simulink model "mdl_Noramlized_LPF_SAR_parallel"  (R2023b)
settings: Solver=VariableStepAuto  StartTime=0.0  StopTime=T_run  FixedStep=1/2.048e6  MaxStep=1e-8  MinStep=1e-12  RelTol=1e-5
undefined symbols (not defined in the file or in its folder): delay, f_s, f_sig, H_matrix, k, NOB, osr, pulse_width, seed_offset, VFS, Vrms
libraries: simulink x9, simulink_extras x8, dspsigops x8
settings Model: Creator=prest  LastModifiedBy=Adyant Balaji
settings DebuggingCC: UnconnectedInputMsg=warning  UnconnectedOutputMsg=warning  UnconnectedLineMsg=warning
settings ModelReferenceCC: EnableRefExpFcnMdlSchedulingChecks=on
settings RTWCC: DLArmComputeVersion=19.05

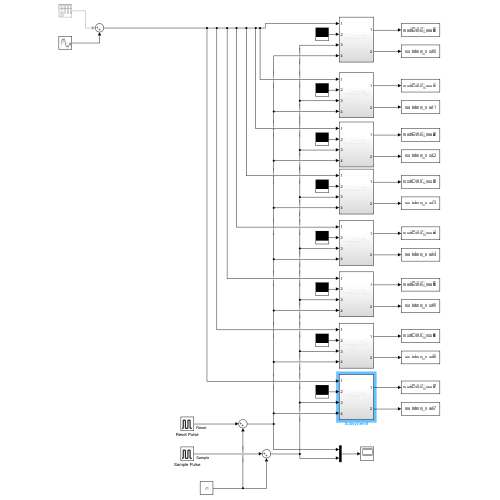
[thumbnail: Simulink's stored preview of the top-level diagram]
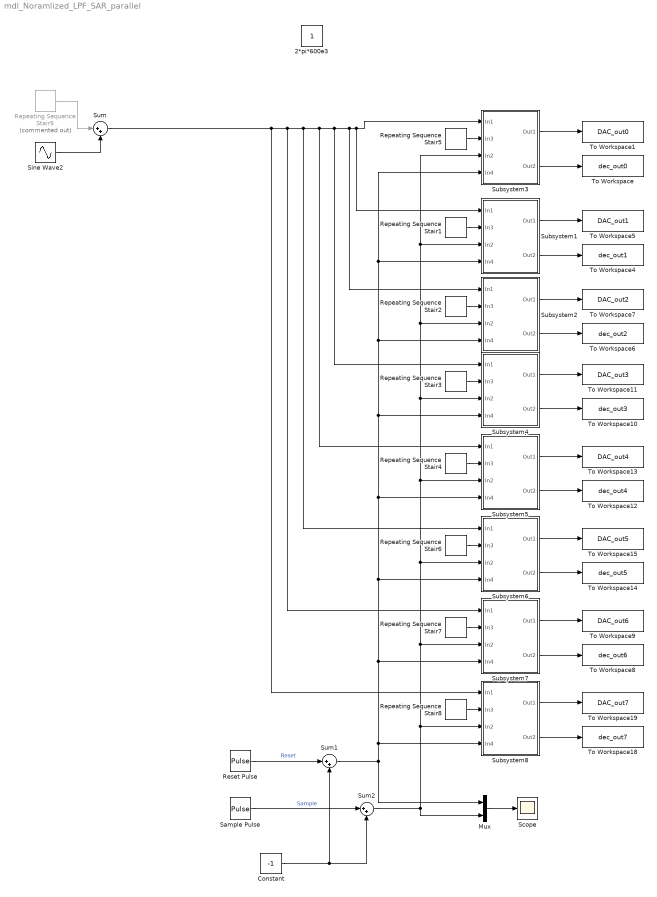
== system mdl_Noramlized_LPF_SAR_parallel ==
  Constant : Constant  Value=-1
  Mux : Mux  Inputs=2
  Repeating Sequence Stair1 : simulink/Sources/Repeating Sequence Stair  OutValues=H_matrix(:, k+1)  tsamp=T_hadamard  OutMin=[]  OutMax=[]  OutDataTypeStr=double  OutputDataTypeScalingMode=double  OutDataType=fixdt(0,8)  ConRadixGroup=Best Precision: Vector-wise  OutScaling=2^-12
  Repeating Sequence Stair2 : simulink/Sources/Repeating Sequence Stair  OutValues=H_matrix(:, k+2)  tsamp=T_hadamard  OutMin=[]  OutMax=[]  OutDataTypeStr=double  OutputDataTypeScalingMode=double  OutDataType=fixdt(0,8)  ConRadixGroup=Best Precision: Vector-wise  OutScaling=2^-12
  Repeating Sequence Stair3 : simulink/Sources/Repeating Sequence Stair  OutValues=H_matrix(:, k+3)  tsamp=T_hadamard  OutMin=[]  OutMax=[]  OutDataTypeStr=double  OutputDataTypeScalingMode=double  OutDataType=fixdt(0,8)  ConRadixGroup=Best Precision: Vector-wise  OutScaling=2^-12
  Repeating Sequence Stair4 : simulink/Sources/Repeating Sequence Stair  OutValues=H_matrix(:, k+4)  tsamp=T_hadamard  OutMin=[]  OutMax=[]  OutDataTypeStr=double  OutputDataTypeScalingMode=double  OutDataType=fixdt(0,8)  ConRadixGroup=Best Precision: Vector-wise  OutScaling=2^-12
  Repeating Sequence Stair5 : simulink/Sources/Repeating Sequence Stair  OutValues=H_matrix(:, k)  tsamp=T_hadamard  OutMin=[]  OutMax=[]  OutDataTypeStr=double  OutputDataTypeScalingMode=double  OutDataType=fixdt(0,8)  ConRadixGroup=Best Precision: Vector-wise  OutScaling=2^-12
  Repeating Sequence Stair6 : simulink/Sources/Repeating Sequence Stair  OutValues=H_matrix(:, k+5)  tsamp=T_hadamard  OutMin=[]  OutMax=[]  OutDataTypeStr=double  OutputDataTypeScalingMode=double  OutDataType=fixdt(0,8)  ConRadixGroup=Best Precision: Vector-wise  OutScaling=2^-12
  Repeating Sequence Stair7 : simulink/Sources/Repeating Sequence Stair  OutValues=H_matrix(:, k+6)  tsamp=T_hadamard  OutMin=[]  OutMax=[]  OutDataTypeStr=double  OutputDataTypeScalingMode=double  OutDataType=fixdt(0,8)  ConRadixGroup=Best Precision: Vector-wise  OutScaling=2^-12
  Repeating Sequence Stair8 : simulink/Sources/Repeating Sequence Stair  OutValues=H_matrix(:, k+7)  tsamp=T_hadamard  OutMin=[]  OutMax=[]  OutDataTypeStr=double  OutputDataTypeScalingMode=double  OutDataType=fixdt(0,8)  ConRadixGroup=Best Precision: Vector-wise  OutScaling=2^-12
  Repeating Sequence Stair9 : simulink/Sources/Repeating Sequence Stair  Commented=on  OutValues=input_sequence  tsamp=T_hadamard  OutMin=[]  OutMax=[]  OutDataTypeStr=double  OutputDataTypeScalingMode=double  OutDataType=fixdt(0,8)  ConRadixGroup=Best Precision: Vector-wise  OutScaling=2^-12
  Reset Pulse : DiscretePulseGenerator  PulseType=Time based  Amplitude=2  Period=osr/f_s  PulseWidth=pulse_width  PhaseDelay=delay
  Sample Pulse : DiscretePulseGenerator  PulseType=Time based  Amplitude=2  Period=osr/f_s  PulseWidth=0.001
  Scope : Scope
  Sine Wave2 : Sin  Amplitude=VFS/2-0.05  Frequency=2*pi*f_sig  SampleTime=0
  Subsystem1 : Subsystem
  Subsystem2 : Subsystem
  Subsystem3 : Subsystem
  Subsystem4 : Subsystem
  Subsystem5 : Subsystem
  Subsystem6 : Subsystem
  Subsystem7 : Subsystem
  Subsystem8 : Subsystem
  Sum : Sum  Inputs=|++
  Sum1 : Sum  Inputs=|++
  Sum2 : Sum  Inputs=|++
  To Workspace : ToWorkspace  VariableName=dec_out0  SampleTime=-1
  To Workspace1 : ToWorkspace  VariableName=DAC_out0  SampleTime=-1
  To Workspace10 : ToWorkspace  VariableName=dec_out3  SampleTime=-1
  To Workspace11 : ToWorkspace  VariableName=DAC_out3  SampleTime=-1
  To Workspace12 : ToWorkspace  VariableName=dec_out4  SampleTime=-1
  To Workspace13 : ToWorkspace  VariableName=DAC_out4  SampleTime=-1
  To Workspace14 : ToWorkspace  VariableName=dec_out5  SampleTime=-1
  To Workspace15 : ToWorkspace  VariableName=DAC_out5  SampleTime=-1
  To Workspace18 : ToWorkspace  VariableName=dec_out7  SampleTime=-1
  To Workspace19 : ToWorkspace  VariableName=DAC_out7  SampleTime=-1
  To Workspace4 : ToWorkspace  VariableName=dec_out1  SampleTime=-1
  To Workspace5 : ToWorkspace  VariableName=DAC_out1  SampleTime=-1
  To Workspace6 : ToWorkspace  VariableName=dec_out2  SampleTime=-1
  To Workspace7 : ToWorkspace  VariableName=DAC_out2  SampleTime=-1
  To Workspace8 : ToWorkspace  VariableName=dec_out6  SampleTime=-1
  To Workspace9 : ToWorkspace  VariableName=DAC_out6  SampleTime=-1
  2*pi*600e3 : Constant  IOType=siggen
  wires:
  Sum/1 -> Subsystem8/1(In1), Subsystem7/1(In1), Subsystem6/1(In1), Subsystem5/1(In1), Subsystem4/1(In1), Subsystem2/1(In1), Subsystem1/1(In1), Subsystem3/1(In1)
  Repeating Sequence Stair5/1 -> Subsystem3/2(In3)
  Subsystem3/1(Out1) -> To Workspace1/1
  Subsystem3/2(Out2) -> To Workspace/1
  Repeating Sequence Stair1/1 -> Subsystem1/2(In3)
  Repeating Sequence Stair8/1 -> Subsystem8/2(In3)
  Subsystem2/2(Out2) -> To Workspace6/1
  Subsystem2/1(Out1) -> To Workspace7/1
  Subsystem1/1(Out1) -> To Workspace5/1
  Subsystem1/2(Out2) -> To Workspace4/1
  Subsystem7/1(Out1) -> To Workspace9/1
  Subsystem7/2(Out2) -> To Workspace8/1
  Subsystem5/1(Out1) -> To Workspace13/1
  Subsystem6/2(Out2) -> To Workspace14/1
  Subsystem6/1(Out1) -> To Workspace15/1
  Subsystem4/2(Out2) -> To Workspace10/1
  Subsystem4/1(Out1) -> To Workspace11/1
  Subsystem5/2(Out2) -> To Workspace12/1
  Subsystem8/2(Out2) -> To Workspace18/1
  Subsystem8/1(Out1) -> To Workspace19/1
  Repeating Sequence Stair2/1 -> Subsystem2/2(In3)
  Repeating Sequence Stair3/1 -> Subsystem4/2(In3)
  Repeating Sequence Stair4/1 -> Subsystem5/2(In3)
  Repeating Sequence Stair6/1 -> Subsystem6/2(In3)
  Repeating Sequence Stair7/1 -> Subsystem7/2(In3)
  Repeating Sequence Stair9/1 -> Sum/1
  Sine Wave2/1 -> Sum/2
  Sample Pulse/1 -> Sum2/1  "Sample"
  Reset Pulse/1 -> Sum1/1  "Reset"
  Constant/1 -> Sum2/2, Sum1/2
  Sum2/1 -> Subsystem8/3(In2), Subsystem7/3(In2), Subsystem6/3(In2), Subsystem5/3(In2), Subsystem4/3(In2), Subsystem2/3(In2), Subsystem1/3(In2), Subsystem3/3(In2), Mux/2
  Sum1/1 -> Subsystem8/4(In4), Subsystem7/4(In4), Subsystem6/4(In4), Subsystem5/4(In4), Subsystem4/4(In4), Subsystem2/4(In4), Subsystem1/4(In4), Subsystem3/4(In4), Mux/1
  Mux/1 -> Scope/1

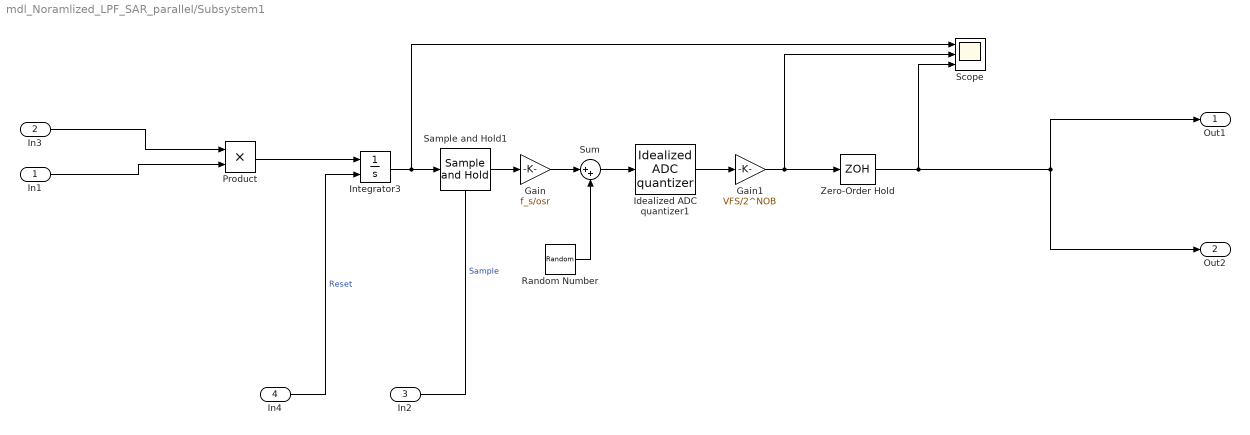
== system mdl_Noramlized_LPF_SAR_parallel/Subsystem1 ==
  In1 : Inport
  In3 : Inport  Port=2
  In2 : Inport  Port=3
  In4 : Inport  Port=4
  Gain : Gain  Gain=f_s/osr
  Gain1 : Gain  Gain=VFS/2^NOB
  Idealized ADC quantizer1 : simulink_extras/Additional Discrete/Idealized ADC quantizer  NumberOfConverterBits=NOB  Vmin=-VFS/2  Vmax=VFS/2  OutputDataType=double  OutputNegativeValues=on
  Integrator3 : Integrator  ExternalReset=falling  ZeroCross=off
  Product : Product
  Random Number : RandomNumber  Variance=(Vrms)^2  Seed=k+1+seed_offset  SampleTime=osr/f_s
  Sample and Hold1 : dspsigops/Sample and Hold  trig=Rising edge  initCond=0  latchinput=off
  Scope : Scope  NumInputPorts=3
  Sum : Sum  Inputs=|++
  Zero-Order Hold : ZeroOrderHold  SampleTime=osr/f_s
  Out1 : Outport
  Out2 : Outport  Port=2
  wires:
  In1/1 -> Product/2
  Zero-Order Hold/1 -> Scope/3, Out2/1, Out1/1
  In3/1 -> Product/1
  Idealized ADC quantizer1/1 -> Gain1/1
  Gain1/1 -> Zero-Order Hold/1, Scope/2
  Product/1 -> Integrator3/1
  Sum/1 -> Idealized ADC quantizer1/1
  Gain/1 -> Sum/1
  Random Number/1 -> Sum/2
  Integrator3/1 -> Sample and Hold1/1, Scope/1
  In4/1 -> Integrator3/2  "Reset"
  Sample and Hold1/1 -> Gain/1
  In2/1 -> Sample and Hold1/Trigger  "Sample"

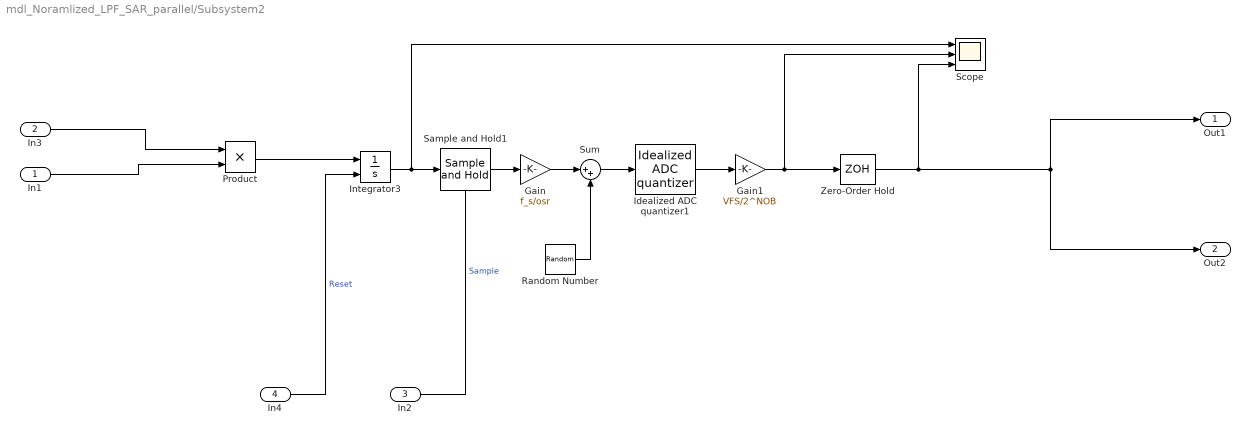
== system mdl_Noramlized_LPF_SAR_parallel/Subsystem2 ==
  In1 : Inport
  In3 : Inport  Port=2
  In2 : Inport  Port=3
  In4 : Inport  Port=4
  Gain : Gain  Gain=f_s/osr
  Gain1 : Gain  Gain=VFS/2^NOB
  Idealized ADC quantizer1 : simulink_extras/Additional Discrete/Idealized ADC quantizer  NumberOfConverterBits=NOB  Vmin=-VFS/2  Vmax=VFS/2  OutputDataType=double  OutputNegativeValues=on
  Integrator3 : Integrator  ExternalReset=falling  ZeroCross=off
  Product : Product
  Random Number : RandomNumber  Variance=(Vrms)^2  Seed=k+2+seed_offset  SampleTime=osr/f_s
  Sample and Hold1 : dspsigops/Sample and Hold  trig=Rising edge  initCond=0  latchinput=off
  Scope : Scope  NumInputPorts=3
  Sum : Sum  Inputs=|++
  Zero-Order Hold : ZeroOrderHold  SampleTime=osr/f_s
  Out1 : Outport
  Out2 : Outport  Port=2
  wires:
  In1/1 -> Product/2
  Zero-Order Hold/1 -> Scope/3, Out2/1, Out1/1
  In3/1 -> Product/1
  Idealized ADC quantizer1/1 -> Gain1/1
  Gain1/1 -> Zero-Order Hold/1, Scope/2
  Product/1 -> Integrator3/1
  Sum/1 -> Idealized ADC quantizer1/1
  Gain/1 -> Sum/1
  Random Number/1 -> Sum/2
  Integrator3/1 -> Sample and Hold1/1, Scope/1
  In4/1 -> Integrator3/2  "Reset"
  Sample and Hold1/1 -> Gain/1
  In2/1 -> Sample and Hold1/Trigger  "Sample"

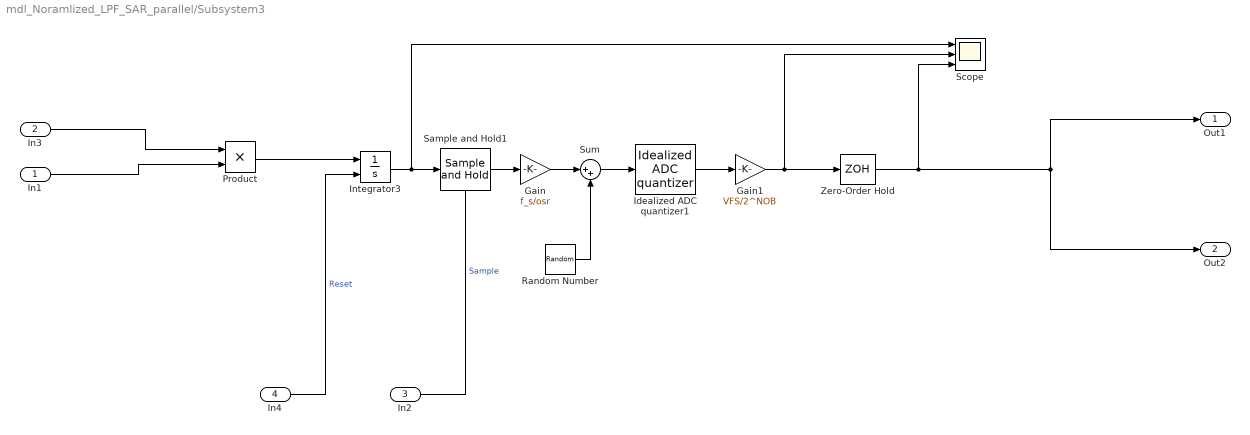
== system mdl_Noramlized_LPF_SAR_parallel/Subsystem3 ==
  In1 : Inport
  In3 : Inport  Port=2
  In2 : Inport  Port=3
  In4 : Inport  Port=4
  Gain : Gain  Gain=f_s/osr
  Gain1 : Gain  Gain=VFS/2^NOB
  Idealized ADC quantizer1 : simulink_extras/Additional Discrete/Idealized ADC quantizer  NumberOfConverterBits=NOB  Vmin=-VFS/2  Vmax=VFS/2  OutputDataType=double  OutputNegativeValues=on
  Integrator3 : Integrator  ExternalReset=falling  ZeroCross=off
  Product : Product
  Random Number : RandomNumber  Variance=(Vrms)^2  Seed=k+seed_offset  SampleTime=osr/f_s
  Sample and Hold1 : dspsigops/Sample and Hold  trig=Rising edge  initCond=0  latchinput=off
  Scope : Scope  NumInputPorts=3
  Sum : Sum  Inputs=|++
  Zero-Order Hold : ZeroOrderHold  SampleTime=osr/f_s
  Out1 : Outport
  Out2 : Outport  Port=2
  wires:
  In1/1 -> Product/2
  Zero-Order Hold/1 -> Scope/3, Out2/1, Out1/1
  In3/1 -> Product/1
  Idealized ADC quantizer1/1 -> Gain1/1
  Gain1/1 -> Zero-Order Hold/1, Scope/2
  Product/1 -> Integrator3/1
  Sum/1 -> Idealized ADC quantizer1/1
  Gain/1 -> Sum/1
  Random Number/1 -> Sum/2
  Integrator3/1 -> Sample and Hold1/1, Scope/1
  In4/1 -> Integrator3/2  "Reset"
  Sample and Hold1/1 -> Gain/1
  In2/1 -> Sample and Hold1/Trigger  "Sample"

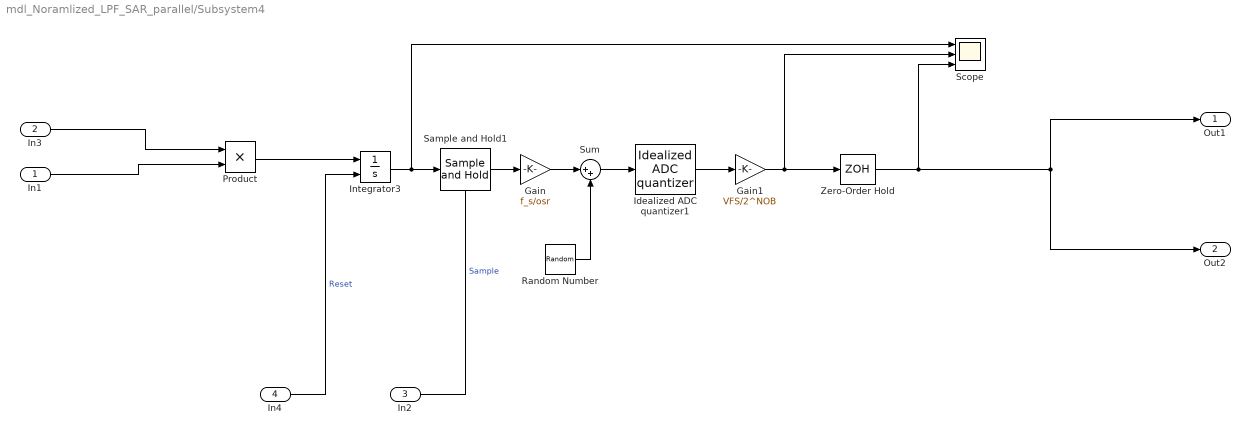
== system mdl_Noramlized_LPF_SAR_parallel/Subsystem4 ==
  In1 : Inport
  In3 : Inport  Port=2
  In2 : Inport  Port=3
  In4 : Inport  Port=4
  Gain : Gain  Gain=f_s/osr
  Gain1 : Gain  Gain=VFS/2^NOB
  Idealized ADC quantizer1 : simulink_extras/Additional Discrete/Idealized ADC quantizer  NumberOfConverterBits=NOB  Vmin=-VFS/2  Vmax=VFS/2  OutputDataType=double  OutputNegativeValues=on
  Integrator3 : Integrator  ExternalReset=falling  ZeroCross=off
  Product : Product
  Random Number : RandomNumber  Variance=(Vrms)^2  Seed=k+3+seed_offset  SampleTime=osr/f_s
  Sample and Hold1 : dspsigops/Sample and Hold  trig=Rising edge  initCond=0  latchinput=off
  Scope : Scope  NumInputPorts=3
  Sum : Sum  Inputs=|++
  Zero-Order Hold : ZeroOrderHold  SampleTime=osr/f_s
  Out1 : Outport
  Out2 : Outport  Port=2
  wires:
  In1/1 -> Product/2
  Zero-Order Hold/1 -> Scope/3, Out2/1, Out1/1
  In3/1 -> Product/1
  Idealized ADC quantizer1/1 -> Gain1/1
  Gain1/1 -> Zero-Order Hold/1, Scope/2
  Product/1 -> Integrator3/1
  Sum/1 -> Idealized ADC quantizer1/1
  Gain/1 -> Sum/1
  Random Number/1 -> Sum/2
  Integrator3/1 -> Sample and Hold1/1, Scope/1
  In4/1 -> Integrator3/2  "Reset"
  Sample and Hold1/1 -> Gain/1
  In2/1 -> Sample and Hold1/Trigger  "Sample"

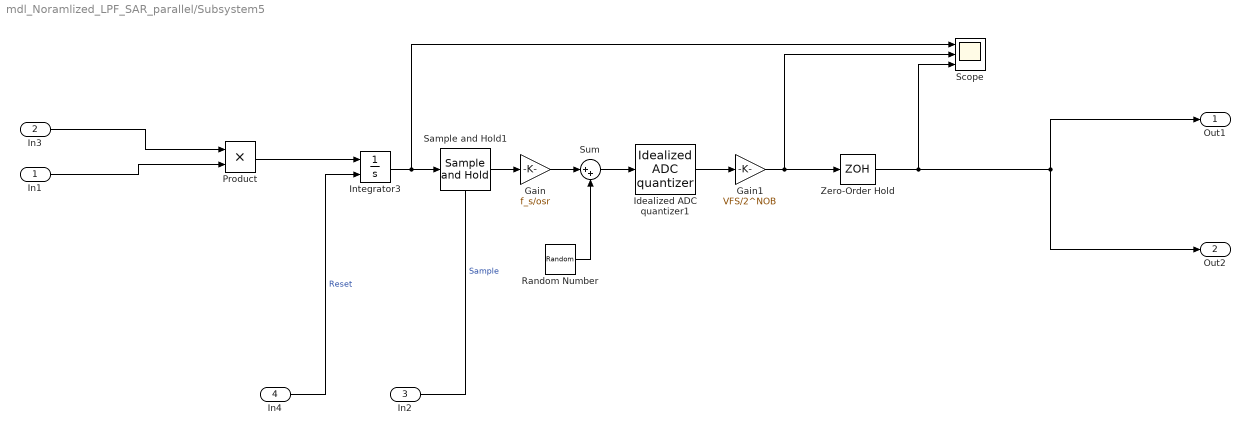
== system mdl_Noramlized_LPF_SAR_parallel/Subsystem5 ==
  In1 : Inport
  In3 : Inport  Port=2
  In2 : Inport  Port=3
  In4 : Inport  Port=4
  Gain : Gain  Gain=f_s/osr
  Gain1 : Gain  Gain=VFS/2^NOB
  Idealized ADC quantizer1 : simulink_extras/Additional Discrete/Idealized ADC quantizer  NumberOfConverterBits=NOB  Vmin=-VFS/2  Vmax=VFS/2  OutputDataType=double  OutputNegativeValues=on
  Integrator3 : Integrator  ExternalReset=falling  ZeroCross=off
  Product : Product
  Random Number : RandomNumber  Variance=(Vrms)^2  Seed=k+4+seed_offset  SampleTime=osr/f_s
  Sample and Hold1 : dspsigops/Sample and Hold  trig=Rising edge  initCond=0  latchinput=off
  Scope : Scope  NumInputPorts=3
  Sum : Sum  Inputs=|++
  Zero-Order Hold : ZeroOrderHold  SampleTime=osr/f_s
  Out1 : Outport
  Out2 : Outport  Port=2
  wires:
  In1/1 -> Product/2
  Zero-Order Hold/1 -> Scope/3, Out2/1, Out1/1
  In3/1 -> Product/1
  Idealized ADC quantizer1/1 -> Gain1/1
  Gain1/1 -> Zero-Order Hold/1, Scope/2
  Product/1 -> Integrator3/1
  Sum/1 -> Idealized ADC quantizer1/1
  Gain/1 -> Sum/1
  Random Number/1 -> Sum/2
  Integrator3/1 -> Sample and Hold1/1, Scope/1
  In4/1 -> Integrator3/2  "Reset"
  Sample and Hold1/1 -> Gain/1
  In2/1 -> Sample and Hold1/Trigger  "Sample"

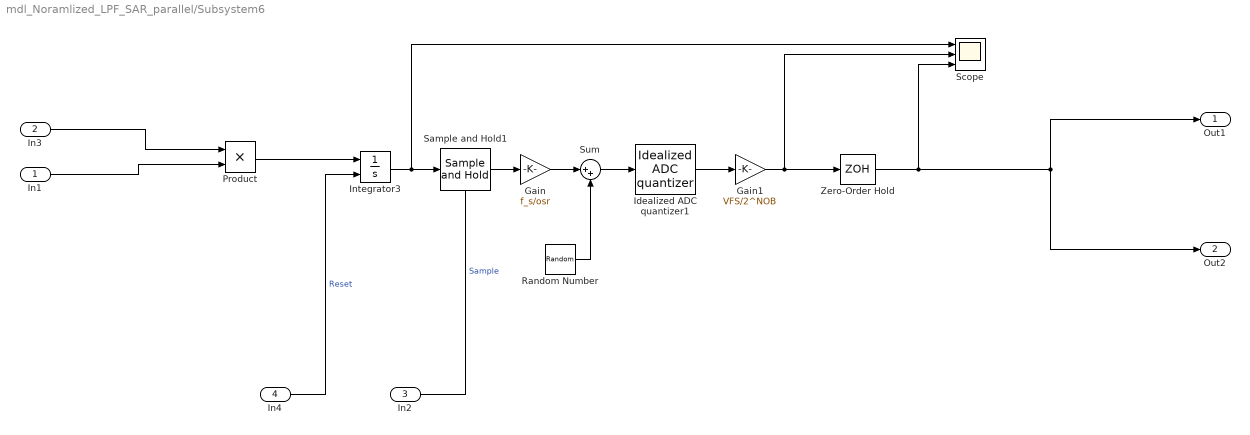
== system mdl_Noramlized_LPF_SAR_parallel/Subsystem6 ==
  In1 : Inport
  In3 : Inport  Port=2
  In2 : Inport  Port=3
  In4 : Inport  Port=4
  Gain : Gain  Gain=f_s/osr
  Gain1 : Gain  Gain=VFS/2^NOB
  Idealized ADC quantizer1 : simulink_extras/Additional Discrete/Idealized ADC quantizer  NumberOfConverterBits=NOB  Vmin=-VFS/2  Vmax=VFS/2  OutputDataType=double  OutputNegativeValues=on
  Integrator3 : Integrator  ExternalReset=falling  ZeroCross=off
  Product : Product
  Random Number : RandomNumber  Variance=(Vrms)^2  Seed=k+5+seed_offset  SampleTime=osr/f_s
  Sample and Hold1 : dspsigops/Sample and Hold  trig=Rising edge  initCond=0  latchinput=off
  Scope : Scope  NumInputPorts=3
  Sum : Sum  Inputs=|++
  Zero-Order Hold : ZeroOrderHold  SampleTime=osr/f_s
  Out1 : Outport
  Out2 : Outport  Port=2
  wires:
  In1/1 -> Product/2
  Zero-Order Hold/1 -> Scope/3, Out2/1, Out1/1
  In3/1 -> Product/1
  Idealized ADC quantizer1/1 -> Gain1/1
  Gain1/1 -> Zero-Order Hold/1, Scope/2
  Product/1 -> Integrator3/1
  Sum/1 -> Idealized ADC quantizer1/1
  Gain/1 -> Sum/1
  Random Number/1 -> Sum/2
  Integrator3/1 -> Sample and Hold1/1, Scope/1
  In4/1 -> Integrator3/2  "Reset"
  Sample and Hold1/1 -> Gain/1
  In2/1 -> Sample and Hold1/Trigger  "Sample"

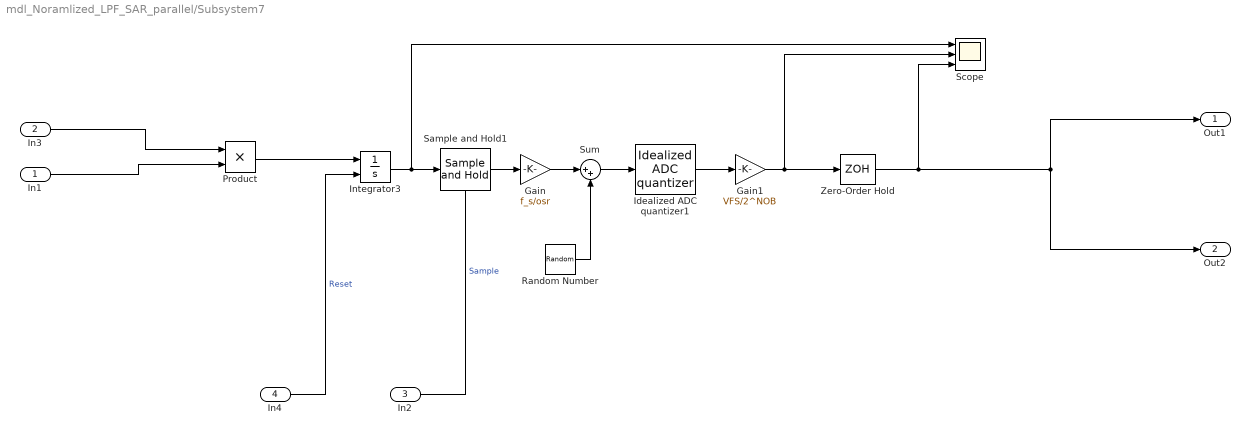
== system mdl_Noramlized_LPF_SAR_parallel/Subsystem7 ==
  In1 : Inport
  In3 : Inport  Port=2
  In2 : Inport  Port=3
  In4 : Inport  Port=4
  Gain : Gain  Gain=f_s/osr
  Gain1 : Gain  Gain=VFS/2^NOB
  Idealized ADC quantizer1 : simulink_extras/Additional Discrete/Idealized ADC quantizer  NumberOfConverterBits=NOB  Vmin=-VFS/2  Vmax=VFS/2  OutputDataType=double  OutputNegativeValues=on
  Integrator3 : Integrator  ExternalReset=falling  ZeroCross=off
  Product : Product
  Random Number : RandomNumber  Variance=(Vrms)^2  Seed=k+6+seed_offset  SampleTime=osr/f_s
  Sample and Hold1 : dspsigops/Sample and Hold  trig=Rising edge  initCond=0  latchinput=off
  Scope : Scope  NumInputPorts=3
  Sum : Sum  Inputs=|++
  Zero-Order Hold : ZeroOrderHold  SampleTime=osr/f_s
  Out1 : Outport
  Out2 : Outport  Port=2
  wires:
  In1/1 -> Product/2
  Zero-Order Hold/1 -> Scope/3, Out2/1, Out1/1
  In3/1 -> Product/1
  Idealized ADC quantizer1/1 -> Gain1/1
  Gain1/1 -> Zero-Order Hold/1, Scope/2
  Product/1 -> Integrator3/1
  Sum/1 -> Idealized ADC quantizer1/1
  Gain/1 -> Sum/1
  Random Number/1 -> Sum/2
  Integrator3/1 -> Sample and Hold1/1, Scope/1
  In4/1 -> Integrator3/2  "Reset"
  Sample and Hold1/1 -> Gain/1
  In2/1 -> Sample and Hold1/Trigger  "Sample"

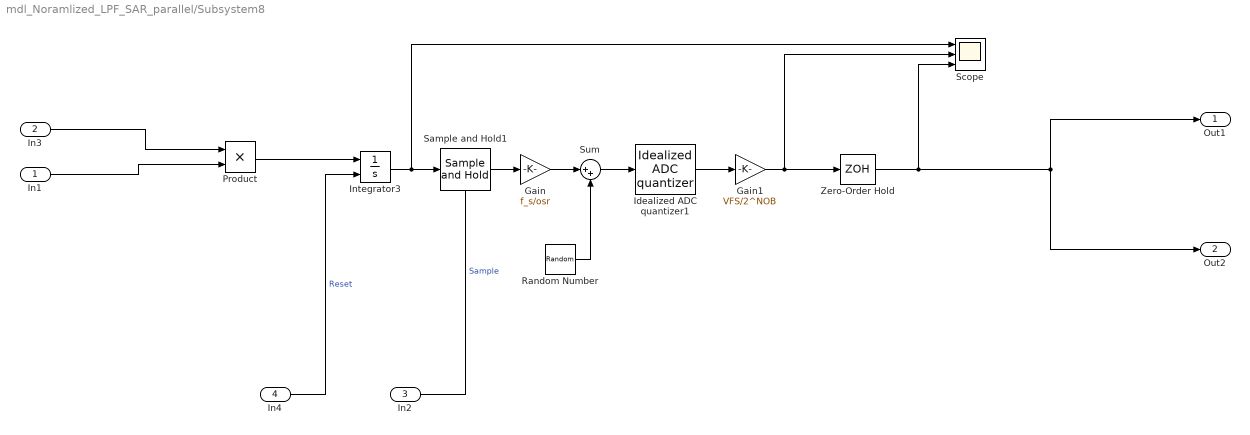
== system mdl_Noramlized_LPF_SAR_parallel/Subsystem8 ==
  In1 : Inport
  In3 : Inport  Port=2
  In2 : Inport  Port=3
  In4 : Inport  Port=4
  Gain : Gain  Gain=f_s/osr
  Gain1 : Gain  Gain=VFS/2^NOB
  Idealized ADC quantizer1 : simulink_extras/Additional Discrete/Idealized ADC quantizer  NumberOfConverterBits=NOB  Vmin=-VFS/2  Vmax=VFS/2  OutputDataType=double  OutputNegativeValues=on
  Integrator3 : Integrator  ExternalReset=falling  ZeroCross=off
  Product : Product
  Random Number : RandomNumber  Variance=(Vrms)^2  Seed=k+7+seed_offset  SampleTime=osr/f_s
  Sample and Hold1 : dspsigops/Sample and Hold  trig=Rising edge  initCond=0  latchinput=off
  Scope : Scope  NumInputPorts=3
  Sum : Sum  Inputs=|++
  Zero-Order Hold : ZeroOrderHold  SampleTime=osr/f_s
  Out1 : Outport
  Out2 : Outport  Port=2
  wires:
  In1/1 -> Product/2
  Zero-Order Hold/1 -> Scope/3, Out2/1, Out1/1
  In3/1 -> Product/1
  Idealized ADC quantizer1/1 -> Gain1/1
  Gain1/1 -> Zero-Order Hold/1, Scope/2
  Product/1 -> Integrator3/1
  Sum/1 -> Idealized ADC quantizer1/1
  Gain/1 -> Sum/1
  Random Number/1 -> Sum/2
  Integrator3/1 -> Sample and Hold1/1, Scope/1
  In4/1 -> Integrator3/2  "Reset"
  Sample and Hold1/1 -> Gain/1
  In2/1 -> Sample and Hold1/Trigger  "Sample"
